simulink library "des_sfun_lib"  (Simulink 7.2)
undefined symbols (not defined in the file or in its folder): des_support
settings Model: Creator=mclune  LastModifiedBy=ywu  ExtModeAutoUpdateStatusClock=off

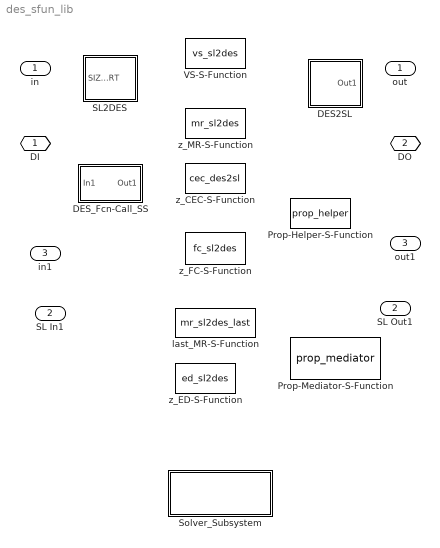
== system des_sfun_lib ==
  in : Inport  PortDimensions=1  DataType=double  OutDataType=sfix(16)  OutScaling=2^0  OutDataTypeStr=double
  SL In1 : Inport  LoadFcn=des_support('desLoadSLPort',gcb,'in')  Port=2  OutDataType=sfix(16)  OutScaling=2^0
      settings: CopyFcn=des_support('desCopySLPort',gcb,'in')  DeleteFcn=des_support('desDeleteSLPort',gcb,'in')  NameChangeFcn=des_support('desNameChangeSLPort',gcb,'in')
  in1 : Inport  Port=3  OutDataType=sfix(16)  OutScaling=2^0
  DES2SL : Subsystem  Opaque=on  mask(msb){PortType=desPortIn, PhysicalDomain=simevents, SubClassName=DES_DES2SL, timingControl=SimEvents, execIndex=0, multipleOutputs=off, attribute=, updateBeforeRead=off, InitValue=0, sampleTime=-1, offsetTime=0, idxBlockMR=0, IsMonitorOnly=off, dimsInfo=1}
      mask prompts: timingControl "Timing Control:"; execIndex "Execution Index:"; multipleOutputs "Allow Multiple Outputs per Time Instant:"; updateBeforeRead "Require update before read"; InitValue "Default value:"; sampleTime "Sample Time:"; offsetTime "Offset Time:"; idxBlockMR "Index of Connected MR Block"; IsMonitorOnly "Is monitor only"; dimsInfo "Dimensions (-1 for inherited)"
      mask help: Transfers data from Entities received in the SimEvents domain to Simulink
      mask init:
      | des_initgateway(gcb, 'out')
      settings: CopyFcn=des_support('desGatewayCopyFcn',gcbh)  NameChangeFcn=des_support('desGatewayNameChangeFcn',gcbh)
      mask Help: web(mech_help('bodysensor'))
      mask StyleString: edit,edit,edit,popup(Simulink|SimEvents|FunctionCall),edit,checkbox,edit,checkbox,edit,edit,edit,edit,checkbox,edit
  DES_Fcn-Call_SS : Subsystem
  Prop-Helper-S-Function : S-Function  FunctionName=prop_helper  Parameters=1, exceptFreeCode  EnableBusSupport=off  mask{InitValue=1, exceptFreeCode=0}
      mask prompts: InitValue "Initial value"; exceptFreeCode "Exception Free Code"
  Prop-Mediator-S-Function : S-Function  FunctionName=prop_mediator  Parameters=num_inports, num_outports, exceptFreeCode  EnableBusSupport=off  mask{num_inports=1, num_outports=1, exceptFreeCode=0}
      mask prompts: num_inports "Number of input ports:"; num_outports "Number of output ports:"; exceptFreeCode "Exception Free Code"
  SL2DES : Subsystem  Opaque=on  mask(msb){PortType=desPortOut, PhysicalDomain=simevents, SubClassName=DES_SL2DES, timingControl=SimEvents, execIndex=1, trigger=None, filter=0, entity=, attribute=, updateBeforeRead=off, InitValue=0, initToFactVal=off, sampleTime=-1, offsetTime=0, idxBlockMR=0, IsMonitorOnly=off, dimsInfo=1}
      mask prompts: timingControl "Timing Control:"; execIndex "Execution Index:"; updateBeforeRead "Require update before read:"; InitValue "Default value:"; initToFactVal "Initialize to Factory Value:"; sampleTime "Sample Time:"; offsetTime "Offset Time:"; idxBlockMR "Index of Connected MR Block"; IsMonitorOnly "Is Monitor only"; dimsInfo "Dimensions (-1 for inherited):"
      mask help: Transfers data from Simulink to Entities created by this block in the SimEvents domain.
      mask init:
      | des_initgateway(gcb, 'in')
      settings: CopyFcn=des_support('desGatewayCopyFcn',gcbh)  NameChangeFcn=des_support('desGatewayNameChangeFcn',gcbh)
      mask Help: web(mech_help('bodyactuator'))
      mask StyleString: edit,edit,edit,popup(Simulink|SimEvents),edit,popup(None|Rising|Falling|Either),edit,edit,edit,checkbox,edit,checkbox,edit,edit,edit,checkbox,edit
  Solver_Subsystem : Subsystem  mask{dumbPara=0}
      mask prompts: dumbPara "dump parameter:"
  VS-S-Function : S-Function  FunctionName=vs_sl2des  Parameters=IsProcessed, numBlocksMR, sl2desCEC_numBlks,des2slCEC_numBlks, numBlocksFC, exceptFreeCode  EnableBusSupport=off  mask{IsProcessed=off, numBlocksMR=-1, sl2desCEC_numBlks=-1, des2slCEC_numBlks=-1, numBlocksFC=-1, exceptFreeCode=0}
      mask prompts: IsProcessed "Is Processed"; numBlocksMR "Number of MR blocks"; sl2desCEC_numBlks "Number of SL to DES CEC blocks"; des2slCEC_numBlks "Number of DES to SL CEC blocks"; numBlocksFC "Number of FC blocks"; exceptFreeCode "Exception Free Code"
  last_MR-S-Function : S-Function  FunctionName=mr_sl2des_last  Parameters=IsProcessed,numInPorts,numOutPorts,numInPortsSL,numOutPortsSL,idxBlockMR, exceptFreeCode  EnableBusSupport=off  mask{IsProcessed=off, numInPorts=-1, numOutPorts=-1, numInPortsSL=-1, numOutPortsSL=-1, idxBlockMR=-1, exceptFreeCode=0}
      mask prompts: IsProcessed "Is Processed"; numInPorts "Number of Input Ports:"; numOutPorts "Number of Output Ports:"; numInPortsSL "Number of Simulink Input Ports:"; numOutPortsSL "Number of Simulink Output Ports:"; idxBlockMR "MR Block Index"; exceptFreeCode "Exception Free Code"
  z_CEC-S-Function : S-Function  FunctionName=cec_des2sl  Parameters=IsProcessed, numInPorts, numOutPorts, idxBlockCEC, dimsInfo, exceptFreeCode  EnableBusSupport=off  mask{IsProcessed=off, numInPorts=-1, numOutPorts=-1, idxBlockCEC=-1, dimsInfo=0, exceptFreeCode=0}
      mask prompts: IsProcessed "Is Processed"; numInPorts "Number of Input Ports"; numOutPorts "Number of Output Ports"; idxBlockCEC "CEC Block Index"; dimsInfo "Dimensions (-1 for inherited):"; exceptFreeCode "Exception Free Code"
  z_ED-S-Function : S-Function  FunctionName=ed_sl2des  Parameters=IsProcessed, numInPorts, numOutPorts, idxBlockCEC, dimsInfo, exceptFreeCode  EnableBusSupport=off  mask{IsProcessed=off, numInPorts=-1, numOutPorts=-1, idxBlockCEC=-1, dimsInfo=0, exceptFreeCode=0}
      mask prompts: IsProcessed "Is Processed"; numInPorts "Number of Input Ports"; numOutPorts "Number of Output Ports"; idxBlockCEC "CEC Block Index"; dimsInfo "Dimensions (-1 for inherited):"; exceptFreeCode "Exception Free Code"
  z_FC-S-Function : S-Function  FunctionName=fc_sl2des  Parameters=IsProcessed, numElements, idxBlockFC, numInPorts, numOutPorts, exceptFreeCode  EnableBusSupport=off  mask{IsProcessed=off, numElements=1, idxBlockFC=-1, numInPorts=-1, numOutPorts=-1, exceptFreeCode=0}
      mask prompts: IsProcessed "Is Processed"; numElements "Number of Elements:"; idxBlockFC "FC Block Idx"; numInPorts "Number of Input Ports"; numOutPorts "Number of Output Ports"; exceptFreeCode "Exception Free Code"
  z_MR-S-Function : S-Function  FunctionName=mr_sl2des  Parameters=IsProcessed,numInPorts,numOutPorts,numInPortsSL,numOutPortsSL,idxBlockMR,IsMonitorOnly, exceptFreeCode  EnableBusSupport=off  mask{IsProcessed=off, numInPorts=-1, numOutPorts=-1, numInPortsSL=-1, numOutPortsSL=-1, idxBlockMR=-1, IsMonitorOnly=off, exceptFreeCode=0}
      mask prompts: IsProcessed "Is Processed"; numInPorts "Number of Input Ports:"; numOutPorts "Number of Output Ports:"; numInPortsSL "Number of Simulink Input Ports:"; numOutPortsSL "Number of Simulink Output Ports:"; idxBlockMR "MR Block Index"; IsMonitorOnly "Is Monitor only"; exceptFreeCode "Exception Free Code"
  DI : PMIOPort  Port=1  Side=Left
  DO : PMIOPort  Orientation=left  Port=2  Side=Right
  out : Outport  OutDataType=sfix(16)  OutScaling=2^0
  SL Out1 : Outport  LoadFcn=des_support('desLoadSLPort',gcb,'out')  Port=2  OutDataType=sfix(16)  OutScaling=2^0
      settings: CopyFcn=des_support('desCopySLPort',gcb,'out')  DeleteFcn=des_support('desDeleteSLPort',gcb,'out')  NameChangeFcn=des_support('desNameChangeSLPort',gcb,'out')
  out1 : Outport  Port=3  OutDataType=sfix(16)  OutScaling=2^0

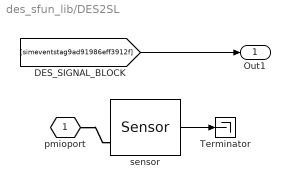
== system des_sfun_lib/DES2SL ==
  Terminator : Terminator
  sensor : Sensor  Tag=__orphan__  PhysicalDomain=simevents  SubClassName=Unknown  PortType=desPortIn
  pmioport : PMIOPort  Port=1  Side=Left
  Out1 : Outport  OutDataType=sfix(16)  OutScaling=2^0
  wires:
  sensor/1 -> Terminator/1
  [simeventstag9ad91986eff3912f] -> Out1/1
  connections:
  pmioport/RConn1 -- sensor/LConn1

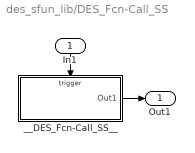
== system des_sfun_lib/DES_Fcn-Call_SS ==
  In1 : Inport  Orientation=down  OutDataType=sfix(16)  OutScaling=2^0
  __DES_Fcn-Call_SS__ : Subsystem  TreatAsAtomicUnit=on
      settings: PropExecContextOutsideSubsystem=on
  Out1 : Outport  OutDataType=sfix(16)  OutScaling=2^0
  wires:
  In1/1 -> __DES_Fcn-Call_SS__/Trigger
  __DES_Fcn-Call_SS__/1(Out1) -> Out1/1

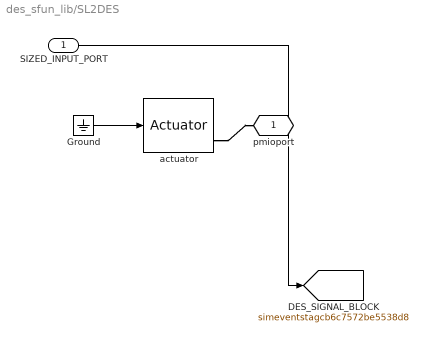
== system des_sfun_lib/SL2DES ==
  SIZED_INPUT_PORT : Inport  OutDataType=sfix(16)  OutScaling=2^0
  Ground : Ground
  actuator : Actuator  Tag=DES_SL2DES  PhysicalDomain=simevents  SubClassName=Unknown  PortType=desPortOut
  pmioport : PMIOPort  Orientation=left  Port=1  Side=Right
  tag scope: simeventstagcb6c7572be5538d8=global
  wires:
  Ground/1 -> actuator/1
  SIZED_INPUT_PORT/1 -> [simeventstagcb6c7572be5538d8]
  connections:
  actuator/RConn1 -- pmioport/RConn1

== system des_sfun_lib/Solver_Subsystem ==

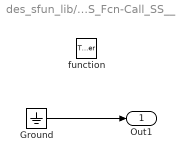
== system des_sfun_lib/DES_Fcn-Call_SS/__DES_Fcn-Call_SS__ ==
  function : TriggerPort  TriggerType=function-call
  Ground : Ground
  Out1 : Outport  OutDataType=sfix(16)  OutScaling=2^0
  wires:
  Ground/1 -> Out1/1
